simulink model "DA42_Model"  (Simulink 7.5)
settings: Solver=ode45  StartTime=0.0  StopTime=inf  RelTol=1e-3
undefined symbols (not defined in the file or in its folder): BHP_A, BHP_B, CP_norm, Pr_Alt, PropEff_norm, S
libraries: simulink_extras x4, aerolibatmos2 x2
(part 2 of 3)

== system DA42_Model/Actuators/Aileron Control Model/Surface Deflection ==
  Aileron Control : Inport
  Aileron Surface (deg) : Lookup  InputValues=|  Table=|
      InputValues=|
      | [-34.2639	
      | -34.0792	
      | -34.0028	
      | -33.7442	
      | -32.3571	
      | -30.4576	
      | -29.1666	
      | -27.9111	
      | -26.4859	
      | -25.2525	
      | -23.9469	
      | -22.3074	
      | -20.7949	
      | -19.4647	
      | -18.0205	
      | -16.5859	
      | -15.2459	
      | -14.0679	
      | -12.8024	
      | -11.4739	
      | -10.0745	
      | -8.4544	
      | -6.9546	
      | -5.2682	
      | -3.2363	
      | -1.6426	
      | -0.9365	
      | -0.4774	
      | -0.0855	
      | 0.1492	
      | 0.9428	
      | 1.6553	
      | 2.656	
      | 4.0557	
      | 5.3005	
      | 6.1849	
      | 7.0228	
      | 7.7845	
      | 8.7125	
      | 9.4451	
      | 10.2121	
      | 11.3116	
      | 12.2433	
      | 13.1013	
      | 14.1017	
      | 15.1219	
      | 16.369	
      | 17.7577	
      | 19.4233	
      | 21.175	
      | 22.7375	
      | 24.384	
      | 26.3066	
      | 27.9061	
      | 29.5096	
      | 31.3812	
      | 33.3818	
      | 34.7307	
      | 35.1717	
      | 35.5534	
      | 36.2978	
      | 37.3223]
      Table=|
      | [-12.0049	
      | -12.007	
      | -12.0296	
      | -11.9474	
      | -11.6142	
      | -11.141	
      | -10.7082	
      | -10.2842	
      | -9.8379	
      | -9.4054	
      | -8.9518	
      | -8.4342	
      | -7.9092	
      | -7.4063	
      | -6.8876	
      | -6.3654	
      | -5.8702	
      | -5.4035	
      | -4.9231	
      | -4.4058	
      | -3.8335	
      | -3.195	
      | -2.5212	
      | -1.8114	
      | -1.1058	
      | -0.5585	
      | -0.2372	
      | -0.0238	
      | 0.1274	
      | 0.2808	
      | 0.667	
      | 1.1152	
      | 1.5066	
      | 1.9716	
      | 2.4846	
      | 2.9171	
      | 3.2324	
      | 3.5469	
      | 3.9018	
      | 4.2252	
      | 4.5692	
      | 4.9412	
      | 5.2802	
      | 5.625	
      | 5.9922	
      | 6.3924	
      | 6.8452	
      | 7.3404	
      | 7.9034	
      | 8.5109	
      | 9.1092	
      | 9.6976	
      | 10.2884	
      | 10.8326	
      | 11.3632	
      | 11.9226	
      | 12.4488	
      | 12.7868	
      | 12.8917	
      | 12.8994	
      | 12.9338	
      | 12.9942]
  Aileron Surface : Outport
  wires:
  Aileron Surface (deg)/1 -> Aileron Surface/1
  Aileron Control/1 -> Aileron Surface (deg)/1

== system DA42_Model/Actuators/Elevator Control Model/Aero Model ==
  Elevator Surface : Inport
  Dynamic Pressure : Inport  Port=2
  AOA : Inport  Port=3
  Flap Surface : Inport  Port=4
  Ch : Sum
  Ch_AOA1 : Lookup2D  RowIndex=[-2.0520646451882 -1.17165815222867 -0.0510552059809828 0.643671787582403 1.02442028022883 1.24100481897819 1.43789985420488 2.22547999511164 3.05243914306374 4.07629332624253 5.97154288610724]  ColumnIndex=[0 15 30]  Table=[-0.000223880597014926 0.000891941391941392 0.000787545787545788;-0.000505330490405118 0.000441364605543709 0.000347985347985348;-0.000872068230277186 -6.18336886993608e-005 -0.000113006396588487;-0.00107675906183369 -0.000402985074626866 -0.00036996336996337;-0.00123880597014925 -0.000573560767590618 -0.000529437427742512;-0.00135820895522388 -0.000692963752665245 -0.000618356603185319;-0.00123027718550107 -0.000786780383795309 -0.000664990376854783;-0.00146908315565032 -0.00111087420042644 -0.000980413187911787;-0.00171641791044776 -0.00145202558635394 -0.00133699633699634;-0.0020319829424307 -0.00183582089552239 -0.00177655677655678;-0.00266311300639659 -0.00259488272921109 -0.00258241758241758]
  Ch_dele2 : Lookup2D  RowIndex=[-6.82218215038285 -6.43662958429216 -5.59434551683249 -4.37110342521096 -3.42057616359746 -2.68365053380721 -2.23508710697837 -1.94672490401697 -1.54088180355278 -1.16707894786208 -0.92143707126533 -0.66511511307742 -0.462193562845324 -0.239586034274828 -0.0243102176076437 0.16793125103329 0.349492638083058 0.541833871163088 0.995637574348416]  ColumnIndex=[0 15 30]  Table=[0.0105 0.0085 0.0065;0.00993603411513859 0.00805970149253732 0.00608102345415778;0.00870788912579958 0.00693390191897655 0.00498933901918977;0.00713859275053305 0.00563752665245203 0.00294243070362473;0.00584221748400853 0.00447761194029851 0.00174840085287846;0.00468230277185501 0.00355650319829425 0.000656716417910451;0.00410234541577825 0.00263539445628998 7.67590618336918e-005;0.0039048848574821 0.00188486140724947 -0.000434968017057568;0.00342004264392324 0.00144136460554371 -0.00104904051172708;0.00307889125799574 0.000929637526652455 -0.00152665245202558;0.00290831556503199 0.000520255863539449 -0.00179957356076759;0.00271062271062271 0.000110874200426441 -0.00197802197802198;0.00247619047619047 -0.000196162046908314 -0.0022;0.00224175824175824 -0.000571428571428573 -0.00232684;0.00202132196162047 -0.0010989010989011 -0.002351;0.00181663113006397 -0.00132053718821266 -0.00243220199232883;0.00168017057569297 -0.00150915750915751 -0.00250130782207885;0.00154371002132196 -0.00162637362637363 -0.00266216431450047;0.00144136460554371 -0.00168498168498169 -0.0028]
  Hinge Moment : Product  RndMeth=Zero
  Product : Product  RndMeth=Zero
  Wing Area : Constant  Value=S
  Aero Force : Outport
  wires:
  Hinge Moment/1 -> Aero Force/1
  Ch_AOA1/1 -> Ch/2
  AOA/1 -> Ch_AOA1/1
  Ch_dele2/1 -> Ch/1
  Flap Surface/1 -> Ch_AOA1/2, Ch_dele2/2
  Elevator Surface/1 -> Ch_dele2/1
  Dynamic Pressure/1 -> Product/1
  Wing Area/1 -> Product/2
  Ch/1 -> Hinge Moment/2
  Product/1 -> Hinge Moment/1

== system DA42_Model/Actuators/Elevator Control Model/Spring Force ==
  Elevator Surface : Inport
  Trim Position : Inport  Port=2
  Elevator Trim Position (in) : Lookup  InputValues=|  Table=|
      InputValues=|
      | [-15.5463	
      | -15.4912	
      | -15.4193	
      | -14.8587	
      | -13.8903	
      | -12.7673	
      | -11.6585	
      | -10.5491	
      | -9.4214	
      | -8.2959	
      | -7.1569	
      | -5.988	
      | -4.8323	
      | -3.7572	
      | -2.7349	
      | -1.6881	
      | -0.7032	
      | -0.0602	
      | -0.0029	
      | 0.5154	
      | 1.4066	
      | 2.3604	
      | 3.2251	
      | 4.0154	
      | 4.7894	
      | 5.5338	
      | 6.2071	
      | 6.8393	
      | 7.4879	
      | 8.1282	
      | 8.6898	
      | 9.1584	
      | 9.5878	
      | 10.0583	
      | 10.6139	
      | 11.1276	
      | 11.3982	
      | 11.4337]
      Table=|
      | [4.3317	
      | 4.3316	
      | 4.3266	
      | 4.3087	
      | 4.2797	
      | 4.2467	
      | 4.2135	
      | 4.1786	
      | 4.1407	
      | 4.102	
      | 4.0636	
      | 4.0234	
      | 3.9821	
      | 3.944	
      | 3.9079	
      | 3.8686	
      | 3.83	
      | 3.8047	
      | 3.7968	
      | 3.7771	
      | 3.7406	
      | 3.7032	
      | 3.6699	
      | 3.6368	
      | 3.6025	
      | 3.5705	
      | 3.543	
      | 3.5186	
      | 3.4939	
      | 3.4695	
      | 3.448	
      | 3.43	
      | 3.4147	
      | 3.4011	
      | 3.3896	
      | 3.3821	
      | 3.3792	
      | 3.3781]
  Spring Delta (in) : Sum  Inputs=-+
  Spring Force (lbs) : Lookup  InputValues=|  Table=|
      InputValues=|
      | [-0.5492	
      | -0.549	
      | -0.5484	
      | -0.5474	
      | -0.546	
      | -0.5446	
      | -0.5436	
      | -0.5428	
      | -0.5408	
      | -0.5355	
      | -0.5239	
      | -0.5045	
      | -0.4776	
      | -0.4454	
      | -0.4103	
      | -0.3746	
      | -0.3401	
      | -0.308	
      | -0.2784	
      | -0.2503	
      | -0.2221	
      | -0.1922	
      | -0.1595	
      | -0.125	
      | -0.0912	
      | -0.0617	
      | -0.0391	
      | -0.0238	
      | -0.0139	
      | -0.0065	
      | 0.0002	
      | 0.0067	
      | 0.0129	
      | 0.0193	
      | 0.0271	
      | 0.0378	
      | 0.052	
      | 0.0692	
      | 0.0878	
      | 0.1061	
      | 0.1226	
      | 0.1371	
      | 0.1502	
      | 0.1629	
      | 0.1758	
      | 0.1894	
      | 0.204	
      | 0.2193	
      | 0.2351	
      | 0.2513	
      | 0.268	
      | 0.2856	
      | 0.3038	
      | 0.3222	
      | 0.3403	
      | 0.3577	
      | 0.3738	
      | 0.3884	
      | 0.4013	
      | 0.4131	
      | 0.4249	
      | 0.4374	
      | 0.4507	
      | 0.4644	
      | 0.4782	
      | 0.4916	
      | 0.5043	
      | 0.5153	
      | 0.5239	
      | 0.5295	
      | 0.5325	
      | 0.5335	
      | 0.5336]
      Table=|
      | [25.8165	
      | 25.6855	
      | 23.0748	
      | 18.8702	
      | 15.2392	
      | 13.2154	
      | 12.492	
      | 12.2992	
      | 12.1745	
      | 11.9865	
      | 11.6712	
      | 11.2197	
      | 10.6851	
      | 10.1411	
      | 9.6959	
      | 9.4242	
      | 9.323	
      | 9.2395	
      | 8.9912	
      | 8.5602	
      | 8.1027	
      | 7.7263	
      | 7.3927	
      | 6.997	
      | 6.4174	
      | 5.4886	
      | 4.175	
      | 2.7157	
      | 1.4582	
      | 0.5014	
      | -0.3847	
      | -1.4833	
      | -2.8299	
      | -4.1883	
      | -5.2622	
      | -5.8949	
      | -6.1375	
      | -6.0785	
      | -5.8625	
      | -5.8436	
      | -6.275	
      | -6.9632	
      | -7.5443	
      | -7.9373	
      | -8.3729	
      | -8.7852	
      | -8.9378	
      | -8.8835	
      | -8.9264	
      | -9.1401	
      | -9.2943	
      | -9.2617	
      | -9.1404	
      | -9.066	
      | -9.0881	
      | -9.2143	
      | -9.4343	
      | -9.6062	
      | -9.6272	
      | -9.5598	
      | -9.5153	
      | -9.5437	
      | -9.6283	
      | -9.8234	
      | -10.1998	
      | -10.6257	
      | -10.9914	
      | -11.6325	
      | -13.5179	
      | -18.049	
      | -26.4048	
      | -38.6743	
      | -53.5025]
  Spring Force : Outport
  wires:
  Spring Force (lbs)/1 -> Spring Force/1
  Elevator Surface/1 -> Elevator Trim Position (in)/1
  Spring Delta (in)/1 -> Spring Force (lbs)/1
  Trim Position/1 -> Spring Delta (in)/2
  Elevator Trim Position (in)/1 -> Spring Delta (in)/1

== system DA42_Model/Actuators/Elevator Control Model/Surface Defection ==
  Elevator Control : Inport
  Elevator Trim Position : Inport  Port=2
  Elevator Trim Position (in) (Zero Force) : Lookup  InputValues=|  Table=|
      InputValues=|
      | [3.3727	
      | 3.3734	
      | 3.3754	
      | 3.3774	
      | 3.3779	
      | 3.3783	
      | 3.3787	
      | 3.3877	
      | 3.3994	
      | 3.4126	
      | 3.4275	
      | 3.4449	
      | 3.466	
      | 3.4902	
      | 3.5151	
      | 3.539	
      | 3.5655	
      | 3.5969	
      | 3.6313	
      | 3.6647	
      | 3.6976	
      | 3.7341	
      | 3.7727	
      | 3.7953	
      | 3.7973	
      | 3.7982	
      | 3.8011	
      | 3.8264	
      | 3.8655	
      | 3.9052	
      | 3.9412	
      | 3.9788	
      | 4.0201	
      | 4.0604	
      | 4.0991	
      | 4.1379	
      | 4.1757	
      | 4.2107	
      | 4.2439	
      | 4.277	
      | 4.307	
      | 4.3269	
      | 4.3304	
      | 4.332	
      | 4.3328]
      Table=|
      | [-1.7069	
      | -1.6739	
      | -1.7214	
      | -1.7303	
      | -1.7256	
      | -1.7275	
      | -1.6225	
      | -1.5601	
      | -1.4928	
      | -1.4241	
      | -1.3533	
      | -1.2764	
      | -1.1905	
      | -1.096	
      | -0.9981	
      | -0.901	
      | -0.8015	
      | -0.695	
      | -0.5823	
      | -0.465	
      | -0.3418	
      | -0.2161	
      | -0.1046	
      | -0.027	
      | -0.0244	
      | -0.0217	
      | 0.0008	
      | 0.0809	
      | 0.2082	
      | 0.3355	
      | 0.4663	
      | 0.5984	
      | 0.737	
      | 0.8779	
      | 1.0154	
      | 1.1482	
      | 1.2776	
      | 1.4028	
      | 1.5235	
      | 1.6372	
      | 1.7301	
      | 1.7855	
      | 1.8029	
      | 1.8038	
      | 1.8038]
  Elevator Surface (deg) : Lookup  InputValues=|  Table=|
      InputValues=|
      | [-2.5703	
      | -2.5622	
      | -2.5495	
      | -2.5278	
      | -2.4944	
      | -2.4487	
      | -2.3926	
      | -2.3307	
      | -2.2688	
      | -2.2101	
      | -2.1552	
      | -2.1017	
      | -2.0462	
      | -1.986	
      | -1.9199	
      | -1.8489	
      | -1.7776	
      | -1.7109	
      | -1.6495	
      | -1.5905	
      | -1.5316	
      | -1.4736	
      | -1.4187	
      | -1.3668	
      | -1.3156	
      | -1.263	
      | -1.2075	
      | -1.1499	
      | -1.0929	
      | -1.0385	
      | -0.9876	
      | -0.9394	
      | -0.8912	
      | -0.8417	
      | -0.7932	
      | -0.7494	
      | -0.7115	
      | -0.6765	
      | -0.6406	
      | -0.6047	
      | -0.5719	
      | -0.5408	
      | -0.5053	
      | -0.4611	
      | -0.4089	
      | -0.3526	
      | -0.2966	
      | -0.2442	
      | -0.1991	
      | -0.1651	
      | -0.1418	
      | -0.1246	
      | -0.1085	
      | -0.0906	
      | -0.0707	
      | -0.0491	
      | -0.0264	
      | -0.0031	
      | 0.0208	
      | 0.0434	
      | 0.0599	
      | 0.0668	
      | 0.0674	
      | 0.0683	
      | 0.0688	
      | 0.0766	
      | 0.0951	
      | 0.121	
      | 0.149	
      | 0.1778	
      | 0.2107	
      | 0.2537	
      | 0.3133	
      | 0.392	
      | 0.4865	
      | 0.5881	
      | 0.6868	
      | 0.7755	
      | 0.8539	
      | 0.9267	
      | 0.999	
      | 1.0741	
      | 1.1527	
      | 1.2357	
      | 1.3245	
      | 1.4198	
      | 1.5176	
      | 1.6121	
      | 1.7004	
      | 1.7852	
      | 1.8726	
      | 1.9674	
      | 2.0707	
      | 2.1787	
      | 2.2839	
      | 2.381	
      | 2.4713	
      | 2.561	
      | 2.6555	
      | 2.7516	
      | 2.839	
      | 2.9084	
      | 2.9591	
      | 2.9989	
      | 3.036	
      | 3.0735]
      Table=|
      | [15.028
      | 15.005	
      | 14.978	
      | 14.963	
      | 14.9329	
      | 14.8247	
      | 14.6137	
      | 14.3191	
      | 13.9868	
      | 13.6574	
      | 13.3489	
      | 13.0551	
      | 12.7539	
      | 12.4243	
      | 12.0546	
      | 11.6499	
      | 11.238	
      | 10.8497	
      | 10.4882	
      | 10.1338	
      | 9.7736	
      | 9.4149	
      | 9.073	
      | 8.7493	
      | 8.4309	
      | 8.1023	
      | 7.7512	
      | 7.3762	
      | 6.9956	
      | 6.6278	
      | 6.2863	
      | 5.9752	
      | 5.6775	
      | 5.377	
      | 5.0773	
      | 4.7945	
      | 4.5379	
      | 4.3	
      | 4.0604	
      | 3.8203	
      | 3.602	
      | 3.3963	
      | 3.156	
      | 2.8523	
      | 2.4987	
      | 2.1234	
      | 1.7473	
      | 1.3848	
      | 1.0619	
      | 0.8115	
      | 0.6457	
      | 0.548	
      | 0.488	
      | 0.4388	
      | 0.3848	
      | 0.3177	
      | 0.2339	
      | 0.1317	
      | 0.0065	
      | -0.1364	
      | -0.2651	
      | -0.4028	
      | -0.3455	
      | -0.3954	
      | -0.3884	
      | -0.3892	
      | -0.372	
      | -0.3561	
      | -0.3625	
      | -0.4185	
      | -0.5538	
      | -0.8087	
      | -1.2272	
      | -1.818	
      | -2.5376	
      | -3.311	
      | -4.0629	
      | -4.7478	
      | -5.3634	
      | -5.9362	
      | -6.5042	
      | -7.1001	
      | -7.7363	
      | -8.4212	
      | -9.1751	
      | -10.0071	
      | -10.8792	
      | -11.7303	
      | -12.5304	
      | -13.3059	
      | -14.1183	
      | -15.0151	
      | -16.0111	
      | -17.0706	
      | -18.1172	
      | -19.0948	
      | -20.0214	
      | -20.9712	
      | -21.9988	
      | -23.0551	
      | -23.9935	
      | -24.6684	
      | -25.0345	
      | -25.1677	
      | -25.1863	
      | -25.1864]
  Gain : Gain  Gain=-1
  Sum : Sum  Inputs=|+-
  Trim Control Position : Outport
  Elevator Surface : Outport  Port=2
  wires:
  Gain/1 -> Elevator Surface/1
  Elevator Surface (deg)/1 -> Gain/1
  Sum/1 -> Trim Control Position/1
  Elevator Trim Position (in) (Zero Force)/1 -> Sum/2
  Elevator Control/1 -> Elevator Surface (deg)/1, Sum/1
  Elevator Trim Position/1 -> Elevator Trim Position (in) (Zero Force)/1

== system DA42_Model/Actuators/Rudder Control Model/Aero Force ==
  Rudder Surface : Inport
  Dynamic Pressure : Inport  Port=2
  Beta : Inport  Port=3
  Flap Surface : Inport  Port=4
  Ch : Sum  Inputs=+++
  Ch_beta : Lookup2D  RowIndex=[-1.88147529083747 0.0358902274679131 3.68999726398883 5.96267359158111]  ColumnIndex=[0 15 30]  Table=[-0.000904761904761904 -0.000831501831501831 -0.000772893772893773;-1.09890109890104e-005 7.69230769230764e-005 0.000135531135531136;0.00158608058608059 0.00167399267399267 0.00173260073260073;0.00258241758241758 0.00265567765567765 0.00275824175824176]
  Ch_delr : Lookup2D  RowIndex=[-1.01520671343935 -0.000539860278868876 1.01500352393412]  ColumnIndex=[0 15 30]  Table=[-0.00296703296703297 -0.00485714285714286 -0.00692673992673993;-0.00142857142857143 -0.00248351648351648 -0.0033816631130064;0.000197802197802198 -8.79120879120881e-005 0.00213186813186813]
  Constant : Constant  Value=0
  Gain : Gain  Gain=180/pi
  Hinge Moment : Product  RndMeth=Zero
  Product : Product  RndMeth=Zero
  Wing Area : Constant  Value=S
  Aero Force : Outport
  wires:
  Gain/1 -> Ch_beta/1
  Beta/1 -> Gain/1
  Constant/1 -> Ch/3
  Hinge Moment/1 -> Aero Force/1
  Ch_beta/1 -> Ch/2
  Ch_delr/1 -> Ch/1
  Ch/1 -> Hinge Moment/2
  Rudder Surface/1 -> Ch_delr/1
  Flap Surface/1 -> Ch_beta/2, Ch_delr/2
  Dynamic Pressure/1 -> Product/1
  Wing Area/1 -> Product/2
  Product/1 -> Hinge Moment/1

== system DA42_Model/Actuators/Rudder Control Model/Interconnect Force ==
  Rudder Control : Inport
  Aileron Control : Inport  Port=2
  Bungee Delta (in) : Sum  Inputs=-+
  Bungee Force (lbs) : Lookup  InputValues=[-1 0 1]  Table=[10 0 -10]
  Cable Displacement (in) : Lookup  InputValues=|  Table=|
      InputValues=|
      | [-33.4770	
      | -27.7272	
      | -22.1070	
      | -14.5237	
      | -7.2592	
      | -0.0745	
      | 7.0405	
      | 13.6672	
      | 20.0049	
      | 26.1632	
      | 32.4012	
      | 38.8884]
      Table=|
      | [1.082677165	
      | 0.885826772	
      | 0.688976378	
      | 0.492125984	
      | 0.295275591	
      | 0.098425197	
      | -0.098425197	
      | -0.295275591	
      | -0.492125984	
      | -0.688976378	
      | -0.885826772	
      | -1.082677165]
  DeadBand : DeadZone  LowerValue=-1  UpperValue=1  SaturateOnIntegerOverflow=on
  Interconnection Displacement (in) : Lookup  InputValues=|  Table=|
      InputValues=|
      | [-49	
      | -42.5	
      | -32	
      | -23.5	
      | -11.25	
      | 0	
      | 8	
      | 14.5	
      | 20.5	
      | 26	
      | 31.25	
      | 33.5]
      Table=|
      | [-0.86614	
      | -0.7874	
      | -0.59055	
      | -0.3937	
      | -0.19685	
      | 0	
      | 0.19685	
      | 0.3937	
      | 0.59055	
      | 0.7874	
      | 0.98425	
      | 1.082675]
  Bungee Force : Outport
  wires:
  Bungee Force (lbs)/1 -> Bungee Force/1
  Bungee Delta (in)/1 -> DeadBand/1
  DeadBand/1 -> Bungee Force (lbs)/1
  Interconnection Displacement (in)/1 -> Bungee Delta (in)/2
  Rudder Control/1 -> Interconnection Displacement (in)/1
  Cable Displacement (in)/1 -> Bungee Delta (in)/1
  Aileron Control/1 -> Cable Displacement (in)/1

== system DA42_Model/Actuators/Rudder Control Model/Spring Force ==
  Rudder Surface : Inport
  Spring Force (lbs) : Lookup  InputValues=|  Table=|
      InputValues=|
      | [-18.8684	
      | -18.7612	
      | -18.5142	
      | -18.1191	
      | -17.6092	
      | -17.026	
      | -16.3882	
      | -15.6756	
      | -14.8649	
      | -13.9867	
      | -13.1069	
      | -12.2669	
      | -11.472	
      | -10.7103	
      | -9.9656	
      | -9.2238	
      | -8.474	
      | -7.7041	
      | -6.9113	
      | -6.1075	
      | -5.3097	
      | -4.5498	
      | -3.8807	
      | -3.3389	
      | -2.9179	
      | -2.5945	
      | -2.3563	
      | -2.1935	
      | -2.0682	
      | -1.8965	
      | -1.5826	
      | -1.1095	
      | -0.6013	
      | -0.1937	
      | 0.0913	
      | 0.3069	
      | 0.5462	
      | 0.9001	
      | 1.374	
      | 1.8791	
      | 2.331	
      | 2.711	
      | 3.0437	
      | 3.3692	
      | 3.7246	
      | 4.1171	
      | 4.5353	
      | 4.9656	
      | 5.3984	
      | 5.8261	
      | 6.2357	
      | 6.6144	
      | 6.9721	
      | 7.3458	
      | 7.7685	
      | 8.2346	
      | 8.7151	
      | 9.1899	
      | 9.6536	
      | 10.1134	
      | 10.5839	
      | 11.0796	
      | 11.5864	
      | 12.071	
      | 12.5198	
      | 12.943	
      | 13.3563	
      | 13.7665	
      | 14.1688	
      | 14.5353	
      | 15.4752	
      | 15.9905	
      | 16.4801	
      | 16.5055]
      Table=|
      | [-71.9757	
      | -66.3864	
      | -56.6269	
      | -52.2704	
      | -51.049	
      | -49.3693	
      | -48.6571	
      | -47.3631	
      | -45.6882	
      | -44.123	
      | -43.5349	
      | -43.9151	
      | -42.4558	
      | -38.7548	
      | -36.8659	
      | -37.3356	
      | -36.6567	
      | -33.9442	
      | -30.149	
      | -28.9352	
      | -29.2168	
      | -27.7956	
      | -23.7911	
      | -19.5254	
      | -16.5935	
      | -12.3873	
      | -7.0509	
      | -2.3454	
      | -1.119	
      | -0.6146	
      | -0.0585	
      | 0.8186	
      | 1.082	
      | 1.9007	
      | 3.32	
      | 3.3637	
      | 6.206	
      | 8.6433	
      | 9.746	
      | 10.7388	
      | 12.4935	
      | 15.3723	
      | 17.0633	
      | 16.961	
      | 17.0739	
      | 18.6254	
      | 20.3762	
      | 21.2493	
      | 22.0907	
      | 22.9549	
      | 24.099	
      | 25.1618	
      | 26.1673	
      | 26.41	
      | 26.1626	
      | 26.568	
      | 29.2129	
      | 30.0453	
      | 29.1571	
      | 30.4003	
      | 31.9073	
      | 31.8134	
      | 31.4787	
      | 31.0858	
      | 31.8845	
      | 32.0986	
      | 31.8153	
      | 32.7692	
      | 35.3075	
      | 35.7006	
      | 37.1939	
      | 47.1063	
      | 63.8761	
      | 76.7729]
  Pedal Force : Outport
  wires:
  Spring Force (lbs)/1 -> Pedal Force/1
  Rudder Surface/1 -> Spring Force (lbs)/1

== system DA42_Model/Actuators/Rudder Control Model/Surface Deflection ==
  Rudder Control : Inport
  Gain : Gain  Gain=-1
  Rudder Surface (deg) : Lookup  InputValues=|  Table=|
      InputValues=|
      | [-57.72404	
      | -57.64784	
      | -57.6326	
      | -57.59704	
      | -57.59704	
      | -57.5564	
      | -56.25084	
      | -52.7177	
      | -48.9712	
      | -45.58538	
      | -41.7703	
      | -37.35832	
      | -32.83712	
      | -28.61564	
      | -25.19426	
      | -22.4409	
      | -20.19046	
      | -17.66824	
      | -14.44244	
      | -11.56462	
      | -9.83234	
      | -8.64108	
      | -7.37616	
      | -5.95376	
      | -4.58978	
      | -4.11226	
      | -4.02336	
      | -3.4036	
      | -1.2319	
      | 0.32004	
      | 0.97028	
      | 1.41986	
      | 1.74498	
      | 1.86182	
      | 1.86436	
      | 1.99898	
      | 2.54	
      | 3.22834	
      | 3.87096	
      | 4.69138	
      | 5.4864	
      | 6.2103	
      | 7.10184	
      | 8.2042	
      | 9.33704	
      | 10.38098	
      | 11.4046	
      | 12.40028	
      | 13.43914	
      | 14.79042	
      | 16.19504	
      | 17.61998	
      | 19.12874	
      | 20.39366	
      | 21.48332	
      | 22.62632	
      | 23.76932	
      | 24.94534	
      | 26.26614	
      | 27.47264	
      | 28.64612	
      | 29.82976	
      | 30.89148	
      | 31.6865	
      | 32.26308	
      | 32.60344	
      | 32.65932	
      | 32.65932	
      | 32.6898	
      | 32.70758	
      | 32.73298	
      | 32.7787	
      | 32.83204	
      | 32.88284]
      Table=|
      | [18.3399	
      | 18.2979	
      | 18.2892	
      | 18.2641	
      | 18.2872	
      | 18.2548	
      | 17.9609	
      | 17.0689	
      | 15.882	
      | 14.6764	
      | 13.3854	
      | 11.9309	
      | 10.3906	
      | 8.8882	
      | 7.6567	
      | 6.7368	
      | 5.9356	
      | 5.0136	
      | 3.9399	
      | 3.0932	
      | 2.6948	
      | 2.5101	
      | 2.3009	
      | 2.0213	
      | 1.7847	
      | 1.7277	
      | 1.7268	
      | 1.3763	
      | 0.5682	
      | -0.1447	
      | -0.4434	
      | -0.5035	
      | -0.5437	
      | -0.5263	
      | -0.5219	
      | -0.7387	
      | -1.132	
      | -1.4991	
      | -1.8742	
      | -2.3431	
      | -2.7803	
      | -3.1326	
      | -3.5471	
      | -4.1141	
      | -4.6911	
      | -5.2002	
      | -5.7292	
      | -6.2943	
      | -6.8225	
      | -7.4429	
      | -8.1703	
      | -8.9183	
      | -9.6447	
      | -10.2823	
      | -10.8389	
      | -11.3489	
      | -11.8624	
      | -12.4541	
      | -13.1011	
      | -13.7329	
      | -14.35	
      | -14.9167	
      | -15.3959	
      | -15.8298	
      | -16.2387	
      | -16.5424	
      | -16.6513	
      | -16.6519	
      | -16.634	
      | -16.6295	
      | -16.6293	
      | -16.6272	
      | -16.6129	
      | -16.5797]
  Rudder Surface : Outport
  wires:
  Gain/1 -> Rudder Surface/1
  Rudder Surface (deg)/1 -> Gain/1
  Rudder Control/1 -> Rudder Surface (deg)/1

== system DA42_Model/DA42/Aerodynamics/Aero Forces and Moments ==
  dyn(q) : Inport
  CD : Inport  Port=2
  CY : Inport  Port=3
  CL : Inport  Port=4
  State : Inport  Port=5
  Croll : Inport  Port=6
  CM : Inport  Port=7
  CN : Inport  Port=8
  Aerodynamic Forces : Subsystem
  Aerodynamic Moments : Subsystem
  Faero : Outport
  Maero : Outport  Port=2
  wires:
  Aerodynamic Moments/1(Maero) -> Maero/1
  Aerodynamic Forces/1(FaeroBody) -> Faero/1
  CN/1 -> Aerodynamic Moments/4(CN)
  CM/1 -> Aerodynamic Moments/3(CM)
  Croll/1 -> Aerodynamic Moments/2(Croll)
  State/1 -> Aerodynamic Forces/4(State)
  CL/1 -> Aerodynamic Forces/3(CL)
  CY/1 -> Aerodynamic Forces/2(CY)
  CD/1 -> Aerodynamic Forces/1(CD)
  dyn(q)/1 -> Aerodynamic Forces/5(dyn(q)), Aerodynamic Moments/1(dyn(q))

== system DA42_Model/DA42/Aerodynamics/CD ==
  State : Inport
  Bus Selector : BusSelector  OutputSignals=alpha
  Find Drag : Lookup_n-D  NumberOfTableDimensions=1  BreakpointsForDimension1="[-0.0986   -0.0828   -0.0654   -0.0511   -0.0312   -0.0179   -0.0084   -0.0003    0.0017    0.0064    0.0076    0.0099 0.0123    0.0157    0.0191    0.0207    0.0354    0.0487    0.0685    0.0828    0.1002    0.1161]"  Table="[0.0745    0.0652    0.0576    0.0528    0.0505    0.0502    0.0477    0.0475    0.0476    0.0475    0.0439    0.0435 0.0432    0.0432    0.0438    0.0485    0.0502    0.0505    0.0528    0.0576    0.0652    0.0745]"  RndMeth=Simplest  InputSameDT=on
  CD : Outport
  wires:
  Bus Selector/1 -> Find Drag/1  "<alpha>"
  State/1 -> Bus Selector/1
  Find Drag/1 -> CD/1

== system DA42_Model/DA42/Aerodynamics/CL ==
  Controls : Inport
  a&bdot : Inport  Port=2
  State : Inport  Port=3
  "   7" : Terminator
  Bus Selector : BusSelector  OutputSignals=elevator
  Bus Selector1 : BusSelector  OutputSignals=alpha,q,TAS
  Demux2 : Demux  Outputs=2
  Fcn : Fcn  Expr=((u[1]+u[2])*Geom(3))/(2*u[3])
  Find CL : Lookup_n-D  NumberOfTableDimensions=1  BreakpointsForDimension1=[-0.26 0.13 0.533 0.991 2.03 2.474 2.96 3.6 4.059 4.45 5.335 5.38 5.5 5.84 6.19 6.569 7.12 7.54 7.92 8.42 8.71 9.29 9.74 10.34 11.176 12.238 13.249 13.605 13.921 14.753 15.482 15.911 16.682]/57.3  Table=[0.257 0.281 0.316 0.389 0.456 0.501 0.56 0.618 0.666 0.698 0.782 0.785 0.825 0.855 0.869 0.917 0.948 1.02 1.048 1.077 1.087 1.166 1.196 1.251 1.283 1.327 1.317 1.361 1.339 1.3066 1.28 1.244 1.195]  RndMeth=Simplest  InputSameDT=on
  Mux : Mux  Inputs=3
  Sum : Sum  Inputs=+++  SaturateOnIntegerOverflow=on
  cladot : Gain  Gain=liftder(3)  SaturateOnIntegerOverflow=on  OutDataTypeStr=Inherit: Same as input  ParamDataTypeStr=Inherit: Same as input
  clde : Gain  Gain=liftder(5)  SaturateOnIntegerOverflow=on  OutDataTypeStr=Inherit: Same as input  ParamDataTypeStr=Inherit: Same as input
  clq : Gain  Gain=liftder(4)  SaturateOnIntegerOverflow=on  OutDataTypeStr=Inherit: Same as input  ParamDataTypeStr=Inherit: Same as input
  CL : Outport
  wires:
  clde/1 -> Sum/3
  clq/1 -> Mux/2
  cladot/1 -> Mux/1
  Demux2/1 -> cladot/1
  State/1 -> Bus Selector1/1
  a&bdot/1 -> Demux2/1
  Controls/1 -> Bus Selector/1
  Sum/1 -> CL/1
  Demux2/2 -> "   7"/1
  Mux/1 -> Fcn/1
  Find CL/1 -> Sum/1
  Fcn/1 -> Sum/2
  Bus Selector/1 -> clde/1  "<elevator>"
  Bus Selector1/1 -> Find CL/1  "<alpha>"
  Bus Selector1/2 -> clq/1  "<q>"
  Bus Selector1/3 -> Mux/3  "<TAS>"

== system DA42_Model/DA42/Aerodynamics/CM ==
  Controls : Inport
  a&bdot : Inport  Port=2
  State : Inport  Port=3
  "   7" : Terminator
  Bus Selector : BusSelector  OutputSignals=elevator
  Bus Selector1 : BusSelector  OutputSignals=alpha,q,TAS
  Demux2 : Demux  Outputs=2
  Fcn : Fcn  Expr=((u[1]+u[2])*Geom(3))/(2*u[3])
  Mux : Mux  Inputs=3
  Sum : Sum  Inputs=+++  SaturateOnIntegerOverflow=on
  cma : Gain  Gain=pitchder(1)  SaturateOnIntegerOverflow=on  OutDataTypeStr=Inherit: Same as input  ParamDataTypeStr=Inherit: Same as input
  cmadot : Gain  Gain=pitchder(2)  SaturateOnIntegerOverflow=on  OutDataTypeStr=Inherit: Same as input  ParamDataTypeStr=Inherit: Same as input
  cmde : Gain  Gain=pitchder(4)  SaturateOnIntegerOverflow=on  OutDataTypeStr=Inherit: Same as input  ParamDataTypeStr=Inherit: Same as input
  cmq : Gain  Gain=pitchder(3)  SaturateOnIntegerOverflow=on  OutDataTypeStr=Inherit: Same as input  ParamDataTypeStr=Inherit: Same as input
  CM : Outport
  wires:
  cmde/1 -> Sum/3
  Fcn/1 -> Sum/2
  Demux2/1 -> cmadot/1
  cma/1 -> Sum/1
  Mux/1 -> Fcn/1
  cmq/1 -> Mux/2
  cmadot/1 -> Mux/1
  State/1 -> Bus Selector1/1
  a&bdot/1 -> Demux2/1
  Controls/1 -> Bus Selector/1
  Sum/1 -> CM/1
  Demux2/2 -> "   7"/1
  Bus Selector/1 -> cmde/1  "<elevator>"
  Bus Selector1/1 -> cma/1  "<alpha>"
  Bus Selector1/2 -> cmq/1  "<q>"
  Bus Selector1/3 -> Mux/3  "<TAS>"

== system DA42_Model/DA42/Aerodynamics/CN ==
  Controls : Inport
  State : Inport  Port=2
  Bus Selector : BusSelector  OutputSignals=aileron,rudder
  Bus Selector1 : BusSelector  OutputSignals=beta,alpha,p,r,TAS
  Divide : Product  Inputs=**
  Fcn : Fcn  Expr=((u[1]+u[2])*Geom(2))/(2*u[3])
  Find CNp : Lookup_n-D  NumberOfTableDimensions=1  BreakpointsForDimension1=[0 1 2 3 4 5 6 7 8]/57.3  Table=[-0.06 -0.078 -0.085 -0.095 -0.107 -0.119 -0.135 -0.14 -0.15]  RndMeth=Simplest  InputSameDT=on
  Mux : Mux  Inputs=3
  Sum : Sum  Inputs=++++  SaturateOnIntegerOverflow=on
  cnb : Gain  Gain=yawder(1)  SaturateOnIntegerOverflow=on  OutDataTypeStr=Inherit: Same as input  ParamDataTypeStr=Inherit: Same as input
  cnda : Gain  Gain=yawder(4)  SaturateOnIntegerOverflow=on  OutDataTypeStr=Inherit: Same as input  ParamDataTypeStr=Inherit: Same as input
  cndr : Gain  Gain=yawder(5)  SaturateOnIntegerOverflow=on  OutDataTypeStr=Inherit: Same as input  ParamDataTypeStr=Inherit: Same as input
  cnr : Gain  Gain=yawder(3)  SaturateOnIntegerOverflow=on  OutDataTypeStr=Inherit: Same as input  ParamDataTypeStr=Inherit: Same as input
  CN : Outport
  wires:
  cndr/1 -> Sum/4
  cnda/1 -> Sum/3
  Fcn/1 -> Sum/2
  cnr/1 -> Mux/2
  cnb/1 -> Sum/1
  Controls/1 -> Bus Selector/1
  Sum/1 -> CN/1
  Mux/1 -> Fcn/1
  Find CNp/1 -> Divide/1
  Divide/1 -> Mux/1
  Bus Selector/1 -> cnda/1  "<aileron>"
  Bus Selector/2 -> cndr/1  "<rudder>"
  State/1 -> Bus Selector1/1
  Bus Selector1/1 -> cnb/1  "<beta>"
  Bus Selector1/2 -> Find CNp/1  "<alpha>"
  Bus Selector1/3 -> Divide/2  "<p>"
  Bus Selector1/4 -> cnr/1  "<r>"
  Bus Selector1/5 -> Mux/3  "<TAS>"

== system DA42_Model/DA42/Aerodynamics/CY ==
  State : Inport
  Controls : Inport  Port=2
  Bus Selector : BusSelector  OutputSignals=rudder
  Bus Selector1 : BusSelector  OutputSignals=beta
  Sum : Sum  SaturateOnIntegerOverflow=on
  cyb : Gain  Gain=sideder(1)  SaturateOnIntegerOverflow=on  OutDataTypeStr=Inherit: Same as input  ParamDataTypeStr=Inherit: Same as input
  cydr : Gain  Gain=sideder(2)  SaturateOnIntegerOverflow=on  OutDataTypeStr=Inherit: Same as input  ParamDataTypeStr=Inherit: Same as input
  CY : Outport
  wires:
  cydr/1 -> Sum/2
  cyb/1 -> Sum/1
  Controls/1 -> Bus Selector/1
  Sum/1 -> CY/1
  Bus Selector/1 -> cydr/1  "<rudder>"
  State/1 -> Bus Selector1/1
  Bus Selector1/1 -> cyb/1  "<beta>"

== system DA42_Model/DA42/Aerodynamics/Croll ==
  Controls : Inport
  State : Inport  Port=2
  Bus Selector : BusSelector  OutputSignals=aileron,rudder
  Bus Selector1 : BusSelector  OutputSignals=beta,alpha,p,r,TAS
  Divide : Product  Inputs=**
  Fcn1 : Fcn  Expr=((u[1]+u[2])*Geom(2))/(2*u[3])
  Find CLr : Lookup_n-D  NumberOfTableDimensions=1  BreakpointsForDimension1=[0 1 2 3 4 5 6 7 8]/57.3  Table=[0.15 0.25 0.32 0.33 0.35 0.35 0.4 0.42 0.45]  RndMeth=Simplest  InputSameDT=on
  Mux : Mux  Inputs=3
  Sum : Sum  Inputs=++++  SaturateOnIntegerOverflow=on
  clb : Gain  Gain=rollder(1)  SaturateOnIntegerOverflow=on  OutDataTypeStr=Inherit: Same as input  ParamDataTypeStr=Inherit: Same as input
  clda : Gain  Gain=rollder(4)  SaturateOnIntegerOverflow=on  OutDataTypeStr=Inherit: Same as input  ParamDataTypeStr=Inherit: Same as input
  cldr : Gain  Gain=rollder(5)  SaturateOnIntegerOverflow=on  OutDataTypeStr=Inherit: Same as input  ParamDataTypeStr=Inherit: Same as input
  clp : Gain  Gain=rollder(2)  SaturateOnIntegerOverflow=on  OutDataTypeStr=Inherit: Same as input  ParamDataTypeStr=Inherit: Same as input
  Croll : Outport
  wires:
  cldr/1 -> Sum/4
  clda/1 -> Sum/3
  Fcn1/1 -> Sum/2
  clb/1 -> Sum/1
  clp/1 -> Mux/1
  State/1 -> Bus Selector1/1
  Controls/1 -> Bus Selector/1
  Sum/1 -> Croll/1
  Mux/1 -> Fcn1/1
  Find CLr/1 -> Divide/1
  Divide/1 -> Mux/2
  Bus Selector/1 -> clda/1  "<aileron>"
  Bus Selector/2 -> cldr/1  "<rudder>"
  Bus Selector1/1 -> clb/1  "<beta>"
  Bus Selector1/2 -> Find CLr/1  "<alpha>"
  Bus Selector1/3 -> clp/1  "<p>"
  Bus Selector1/5 -> Mux/3  "<TAS>"
  Bus Selector1/4 -> Divide/2  "<r>"

== system DA42_Model/DA42/Equations of motion numerical integration /Flat Earth Navigation ==
  note: 1  roll
      | 2  pitch
      | 3  yaw
      | 4 u
      | 5 v
      | 6 w
  Euler Angles : Inport
  Velocity : Inport  Port=2
  Alt : Integrator  InitialCondition=x0(12)
  Alttitude Dot : Fcn  Expr=u[4] * sin(u[2]) - u[5] * sin(u[1]) * cos(u[2]) - u[6] * cos(u[1]) * cos(u[2])
  Demux : Demux  Outputs=3
  Demux1 : Demux  Outputs=3
  East : Integrator  InitialCondition=x0(11)
  East Dot : Fcn  Expr=u[4] * cos(u[2])* sin(u[3]) + u[5] * (cos(u[1])*cos(u[3]) + sin(u[1])*sin(u[2])*sin(u[3])) + u[6] * (-sin(u[1])*cos(u[3])+cos(u[1])*sin(u[2])*sin(u[3]))
  Mux : Mux  Inputs=6
  Mux1 : Mux  Inputs=3
  North : Integrator  InitialCondition=x0(10)
  North Dot : Fcn  Expr=u[4] * cos(u[2]) * cos(u[3]) + u[5]*(-cos(u[1])*sin(u[3])+sin(u[1])*sin(u[2])*sin(u[3]))+u[6]*(sin(u[1])*sin(u[3])+cos(u[1])*sin(u[2])*cos(u[3]))
  Position : Outport
  wires:
  Mux1/1 -> Position/1
  Alt/1 -> Mux1/3
  North/1 -> Mux1/1
  East/1 -> Mux1/2
  Alttitude Dot/1 -> Alt/1
  North Dot/1 -> North/1
  East Dot/1 -> East/1
  Mux/1 -> North Dot/1, Alttitude Dot/1, East Dot/1
  Demux1/3 -> Mux/6
  Demux1/2 -> Mux/5
  Demux1/1 -> Mux/4
  Demux/3 -> Mux/3
  Demux/2 -> Mux/2
  Demux/1 -> Mux/1
  Velocity/1 -> Demux1/1
  Euler Angles/1 -> Demux/1

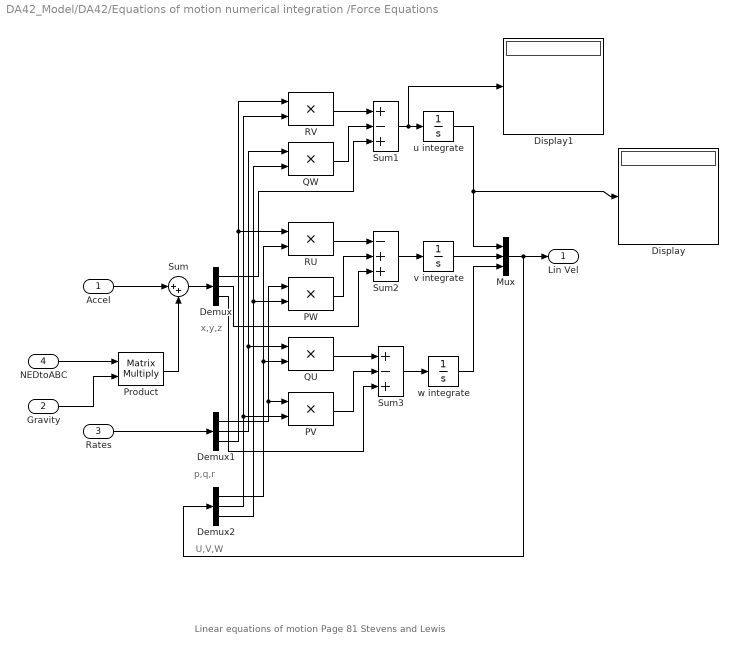
== system DA42_Model/DA42/Equations of motion numerical integration /Force Equations ==
  note: Linear equations of motion
      | Page 81 Stevens and Lewis
  note: x,y,z
  note: p,q,r
  note: U,V,W
  Accel : Inport
  Gravity : Inport  Port=2
  Rates : Inport  Port=3
  NEDtoABC : Inport  Port=4
  Demux : Demux  Outputs=3
  Demux1 : Demux  Outputs=3
  Demux2 : Demux  Outputs=3
  Display : Display
  Display1 : Display
  Mux : Mux  Inputs=3
  PV : Product  SaturateOnIntegerOverflow=on  OutDataTypeStr=Inherit: Same as first input
  PW : Product  SaturateOnIntegerOverflow=on  OutDataTypeStr=Inherit: Same as first input
  Product : Product  Multiplication=Matrix(*)  SaturateOnIntegerOverflow=on  OutDataTypeStr=Inherit: Same as first input
  QU : Product  SaturateOnIntegerOverflow=on  OutDataTypeStr=Inherit: Same as first input
  QW : Product  SaturateOnIntegerOverflow=on  OutDataTypeStr=Inherit: Same as first input
  RU : Product  SaturateOnIntegerOverflow=on  OutDataTypeStr=Inherit: Same as first input
  RV : Product  SaturateOnIntegerOverflow=on  OutDataTypeStr=Inherit: Same as first input
  Sum : Sum  Inputs=|++  SaturateOnIntegerOverflow=on
  Sum1 : Sum  Inputs=+-+  SaturateOnIntegerOverflow=on
  Sum2 : Sum  Inputs=-++  SaturateOnIntegerOverflow=on
  Sum3 : Sum  Inputs=+-+  SaturateOnIntegerOverflow=on
  u integrate : Integrator  InitialCondition=x0(1)
  v integrate : Integrator  InitialCondition=x0(2)
  w integrate : Integrator  InitialCondition=x0(3)
  Lin Vel : Outport
  wires:
  w integrate/1 -> Mux/3
  v integrate/1 -> Mux/2
  u integrate/1 -> Display/1, Mux/1
  Sum3/1 -> w integrate/1
  Sum2/1 -> v integrate/1
  Sum1/1 -> Display1/1, u integrate/1
  Product/1 -> Sum/2
  NEDtoABC/1 -> Product/1
  Gravity/1 -> Product/2
  Demux/3 -> Sum3/3
  PV/1 -> Sum3/2
  QU/1 -> Sum3/1
  Demux/2 -> Sum2/3
  PW/1 -> Sum2/2
  Demux1/1 -> PW/1, PV/1
  RU/1 -> Sum2/1
  Demux2/1 -> QU/2, RU/2
  Demux/1 -> Sum1/3
  QW/1 -> Sum1/2
  Demux2/3 -> PW/2, QW/2
  Demux1/2 -> QU/1, QW/1
  RV/1 -> Sum1/1
  Demux2/2 -> PV/2, RV/2
  Demux1/3 -> RU/1, RV/1
  Mux/1 -> Lin Vel/1, Demux2/1
  Rates/1 -> Demux1/1
  Accel/1 -> Sum/1
  Sum/1 -> Demux/1

== system DA42_Model/DA42/Equations of motion numerical integration /Gravity Model ==
  Constant : Constant  Value=0
  Constant1 : Constant  Value=32.2
  Mux : Mux  Inputs=3
  Gravity : Outport
  wires:
  Mux/1 -> Gravity/1
  Constant1/1 -> Mux/3
  Constant/1 -> Mux/2, Mux/1

== system DA42_Model/DA42/Equations of motion numerical integration /Inert-body ==
  Euler : Inport
  11 : Fcn  Expr=cos(u[2])*cos(u[3])
  12 : Fcn  Expr=-cos(u[1])*sin(u[3])+sin(u[1])*sin(u[2])*cos(u[3])
  13 : Fcn  Expr=sin(u[1])*sin(u[3])+cos(u[1])*sin(u[2])*cos(u[3])
  21 : Fcn  Expr=cos(u[2])*sin(u[3])
  22 : Fcn  Expr=cos(u[1])*cos(u[3]) + sin(u[1])*sin(u[2])*sin(u[3])
  23 : Fcn  Expr=-sin(u[1])*cos(u[3])+cos(u[1])*sin(u[2])*sin(u[3])
  31 : Fcn  Expr=-sin(u[2])
  32 : Fcn  Expr=sin(u[1]) * cos(u[2])
  33 : Fcn  Expr=cos(u[1])*cos(u[2])
  Matrix Concatenation : Concatenate  NumInputs=3  Mode=Multidimensional array
  Matrix Concatenation1 : Concatenate  NumInputs=3  Mode=Multidimensional array
  Matrix Concatenation2 : Concatenate  NumInputs=3  Mode=Multidimensional array
  Matrix Concatenation3 : Concatenate  NumInputs=3  Mode=Multidimensional array  ConcatenateDimension=2
  NEDtoBC : Outport
  wires:
  Matrix Concatenation3/1 -> NEDtoBC/1
  Matrix Concatenation2/1 -> Matrix Concatenation3/3
  Matrix Concatenation/1 -> Matrix Concatenation3/1
  Matrix Concatenation1/1 -> Matrix Concatenation3/2
  33/1 -> Matrix Concatenation2/3
  31/1 -> Matrix Concatenation2/1
  32/1 -> Matrix Concatenation2/2
  23/1 -> Matrix Concatenation1/3
  21/1 -> Matrix Concatenation1/1
  22/1 -> Matrix Concatenation1/2
  13/1 -> Matrix Concatenation/3
  11/1 -> Matrix Concatenation/1
  12/1 -> Matrix Concatenation/2
  Euler/1 -> 32/1, 33/1, 31/1, 23/1, 22/1, 21/1, 13/1, 12/1, 11/1

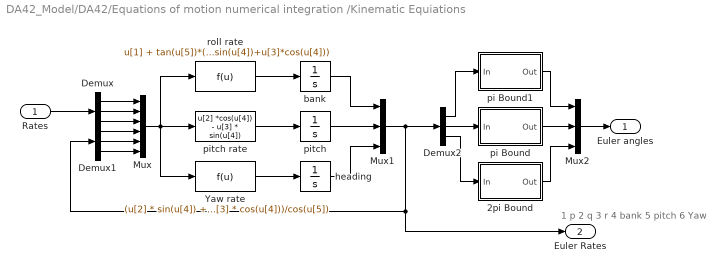
== system DA42_Model/DA42/Equations of motion numerical integration /Kinematic Equiations ==
  note: 1  p
      | 2  q
      | 3  r
      | 4  bank
      | 5 pitch
      | 6 Yaw
  Rates : Inport
  2pi Bound : Subsystem
      mask Type: 2pi bound
      mask Description: Bounds the input angle to [0, 2pi]. When 0 bound is exceeded the output wraps back to 2pi; when the 2pi bound is exceeded the output wraps back to 0.
      mask Help:
      | Bounds the input angle to [0, 2pi]. When 0 bound is exceeded the output wraps back to 2pi; when the 2pi bound is exceeded the output wraps back to 0.
      | <P><B>Input:</B> any angle in radians, from -Inf to Inf;</P>
      | <P><B>Output:</B> an angle in radians between zero and 2pi.</P>
  Demux : Demux  Outputs=3
  Demux1 : Demux  Outputs=3
  Demux2 : Demux  Outputs=3
  Mux : Mux  Inputs=6
  Mux1 : Mux  Inputs=3
  Mux2 : Mux  Inputs=3
  Yaw rate : Fcn  Expr=(u[2] * sin(u[4]) + u[3] * cos(u[4]))/cos(u[5])
  bank : Integrator  InitialCondition=x0(7)
  heading : Integrator  InitialCondition=x0(9)
  pi Bound : Subsystem
      mask Type: pi bound
      mask Description: Bounds the input angle to [-pi, pi]. When -pi bound is exceeded the output wraps back to pi; when the pi bound is exceeded the output wraps back to -pi.
      mask Help:
      | Bounds the input angle to [-pi, pi]. When -pi bound is exceeded the output wraps back to pi; when the pi bound is exceeded the output wraps back to -pi.
      | <P><B>Input:</B> any angle in radians, from -Inf to Inf;</P>
      | <P><B>Output:</B> an angle in radians between -pi and pi.</P>
  pi Bound1 : Subsystem
      mask Type: pi bound
      mask Description: Bounds the input angle to [-pi, pi]. When -pi bound is exceeded the output wraps back to pi; when the pi bound is exceeded the output wraps back to -pi.
      mask Help:
      | Bounds the input angle to [-pi, pi]. When -pi bound is exceeded the output wraps back to pi; when the pi bound is exceeded the output wraps back to -pi.
      | <P><B>Input:</B> any angle in radians, from -Inf to Inf;</P>
      | <P><B>Output:</B> an angle in radians between -pi and pi.</P>
  pitch : Integrator  InitialCondition=x0(8)
  pitch rate : Fcn  Expr=u[2] *cos(u[4]) - u[3] * sin(u[4])
  roll rate : Fcn  Expr=u[1] + tan(u[5])*(u[2]*sin(u[4])+u[3]*cos(u[4]))
  Euler angles : Outport
  Euler Rates : Outport  Port=2
  wires:
  Mux1/1 -> Euler Rates/1, Demux1/1, Demux2/1
  heading/1 -> Mux1/3
  pitch/1 -> Mux1/2
  bank/1 -> Mux1/1
  Yaw rate/1 -> heading/1
  roll rate/1 -> bank/1
  pitch rate/1 -> pitch/1
  2pi Bound/1(Out) -> Mux2/3
  pi Bound1/1(Out) -> Mux2/1
  pi Bound/1(Out) -> Mux2/2
  Mux2/1 -> Euler angles/1
  Demux2/1 -> pi Bound1/1(In)
  Demux2/2 -> pi Bound/1(In)
  Demux2/3 -> 2pi Bound/1(In)
  Mux/1 -> pitch rate/1, Yaw rate/1, roll rate/1
  Demux/1 -> Mux/1
  Demux1/3 -> Mux/6
  Demux1/2 -> Mux/5
  Demux1/1 -> Mux/4
  Demux/3 -> Mux/3
  Demux/2 -> Mux/2
  Rates/1 -> Demux/1

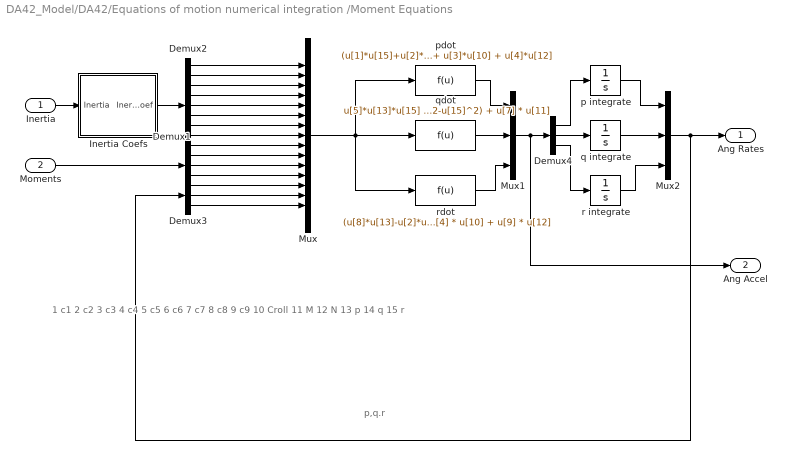
== system DA42_Model/DA42/Equations of motion numerical integration /Moment Equations ==
  note: p,q.r
  note: 1   c1
      | 2   c2
      | 3   c3
      | 4  c4
      | 5  c5
      | 6  c6
      | 7  c7
      | 8  c8
      | 9  c9
      | 10 Croll
      | 11  M
      | 12  N
      | 13  p
      | 14  q
      | 15  r
  Inertia : Inport
  Moments : Inport  Port=2
  Demux1 : Demux  Outputs=3
  Demux2 : Demux  Outputs=9
  Demux3 : Demux  Outputs=3
  Demux4 : Demux  Outputs=3
  Inertia Coefs : Subsystem
  Mux : Mux  Inputs=15
  Mux1 : Mux  Inputs=3
  Mux2 : Mux  Inputs=3
  p integrate : Integrator  InitialCondition=x0(4)
  pdot : Fcn  Expr=(u[1]*u[15]+u[2]*u[13])*u[14] + u[3]*u[10] + u[4]*u[12]
  q integrate : Integrator  InitialCondition=x0(5)
  qdot : Fcn  Expr=u[5]*u[13]*u[15] - u[6]*(u[13]^2-u[15]^2) + u[7] * u[11]
  r integrate : Integrator  InitialCondition=x0(6)
  rdot : Fcn  Expr=(u[8]*u[13]-u[2]*u[15]) * u[14] + u[4] * u[10] + u[9] * u[12]
  Ang Rates : Outport
  Ang Accel : Outport  Port=2
  wires:
  r integrate/1 -> Mux2/3
  q integrate/1 -> Mux2/2
  p integrate/1 -> Mux2/1
  Mux2/1 -> Demux3/1, Ang Rates/1
  Demux4/3 -> r integrate/1
  Demux4/2 -> q integrate/1
  Demux4/1 -> p integrate/1
  Mux1/1 -> Demux4/1, Ang Accel/1
  rdot/1 -> Mux1/3
  pdot/1 -> Mux1/1
  qdot/1 -> Mux1/2
  Mux/1 -> rdot/1, qdot/1, pdot/1
  Demux3/3 -> Mux/15
  Demux3/2 -> Mux/14
  Demux3/1 -> Mux/13
  Demux1/3 -> Mux/12
  Demux1/2 -> Mux/11
  Demux1/1 -> Mux/10
  Demux2/9 -> Mux/9
  Demux2/8 -> Mux/8
  Demux2/7 -> Mux/7
  Demux2/6 -> Mux/6
  Demux2/5 -> Mux/5
  Demux2/4 -> Mux/4
  Demux2/3 -> Mux/3
  Demux2/2 -> Mux/2
  Demux2/1 -> Mux/1
  Inertia Coefs/1(Iner Coef) -> Demux2/1
  Moments/1 -> Demux1/1
  Inertia/1 -> Inertia Coefs/1(Inertia)

== system DA42_Model/DA42/Linear Accelerations and Moments/Cross Prod Moment due Leng ==
  Vec 1 : Inport
  Vec 2 : Inport  Port=2
  Check prob not zero : Constant  Value=0
  Demux : Demux  Outputs=3
  J axis : Fcn  Expr=u[4]*u[3] - u[6]*u[1]
  Mux : Mux  Inputs=6
  Mux1 : Mux  Inputs=3
  i axis : Fcn  Expr=u[6]*u[2] - u[5]*u[3]
  k axis : Fcn  Expr=u[5]*u[1] - u[4]*u[2]
  X Prod : Outport
  wires:
  Mux1/1 -> X Prod/1
  k axis/1 -> Mux1/3
  i axis/1 -> Mux1/1
  J axis/1 -> Mux1/2
  Mux/1 -> k axis/1, J axis/1, i axis/1
  Demux/2 -> Mux/2
  Demux/3 -> Mux/3
  Check prob not zero/1 -> Mux/6, Mux/5
  Demux/1 -> Mux/1
  Vec 1/1 -> Demux/1
  Vec 2/1 -> Mux/4

== system DA42_Model/DA42/Linear Accelerations and Moments/Cross Prod Moment due Reng ==
  Vec 1 : Inport
  Vec 2 : Inport  Port=2
  Check prob not zero : Constant  Value=0
  Demux : Demux  Outputs=3
  J axis : Fcn  Expr=u[4]*u[3] - u[6]*u[1]
  Mux : Mux  Inputs=6
  Mux1 : Mux  Inputs=3
  i axis : Fcn  Expr=u[6]*u[2] - u[5]*u[3]
  k axis : Fcn  Expr=u[5]*u[1] - u[4]*u[2]
  X Prod : Outport
  wires:
  Mux1/1 -> X Prod/1
  k axis/1 -> Mux1/3
  i axis/1 -> Mux1/1
  J axis/1 -> Mux1/2
  Mux/1 -> k axis/1, J axis/1, i axis/1
  Demux/2 -> Mux/2
  Demux/3 -> Mux/3
  Check prob not zero/1 -> Mux/6, Mux/5
  Demux/1 -> Mux/1
  Vec 1/1 -> Demux/1
  Vec 2/1 -> Mux/4

== system DA42_Model/DA42/Linear Accelerations and Moments/Cross Prod Moment due to Aero ==
  Vec 1 : Inport
  Vec 2 : Inport  Port=2
  Demux : Demux  Outputs=3
  Demux1 : Demux  Outputs=3
  J axis : Fcn  Expr=u[4]*u[3] - u[6]*u[1]
  Mux : Mux  Inputs=6
  Mux1 : Mux  Inputs=3
  i axis : Fcn  Expr=u[6]*u[2] - u[5]*u[3]
  k axis : Fcn  Expr=u[5]*u[1] - u[4]*u[2]
  X Prod : Outport
  wires:
  Mux1/1 -> X Prod/1
  k axis/1 -> Mux1/3
  i axis/1 -> Mux1/1
  J axis/1 -> Mux1/2
  Mux/1 -> k axis/1, J axis/1, i axis/1
  Demux/2 -> Mux/2
  Demux/3 -> Mux/3
  Demux1/1 -> Mux/4
  Demux1/2 -> Mux/5
  Demux1/3 -> Mux/6
  Demux/1 -> Mux/1
  Vec 1/1 -> Demux/1
  Vec 2/1 -> Demux1/1

== system DA42_Model/DA42/Linear Accelerations and Moments/Thrust Components ==
  Feng : Inport
  Bus Selector : BusSelector  OutputSignals=L_Thrust,R_Thrust
  Sum : Sum  Inputs=|++
  X Percent : Gain  Gain=thrustPercent(1)
  Y Percent : Gain  Gain=thrustPercent(2)
  Z Percent : Gain  Gain=thrustPercent(3)
  X% : Outport
  Y% : Outport  Port=2
  Z% : Outport  Port=3
  wires:
  Sum/1 -> Z Percent/1, Y Percent/1, X Percent/1
  Bus Selector/2 -> Sum/2  "<R_Thrust>"
  Bus Selector/1 -> Sum/1  "<L_Thrust>"
  Feng/1 -> Bus Selector/1
  Z Percent/1 -> Z%/1
  Y Percent/1 -> Y%/1
  X Percent/1 -> X%/1
